simulink model "ex3_sim2m"  (R2022b)
settings: Solver=ode45  StartTime=0.0  StopTime=5  MaxStep=0.0001  RelTol=1e-3
undefined symbols (not defined in the file): d0, denD, DiscIntNeverNeededParam, mot, numD, pid, r, rad2pulse, Ts, umax
settings Model: Creator=loren  LastModifiedBy=loren
settings DataIOCC: ReturnWorkspaceOutputs=off

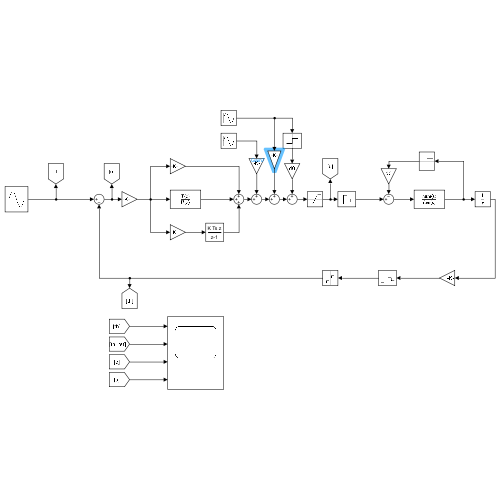
[thumbnail: Simulink's stored preview of the top-level diagram]
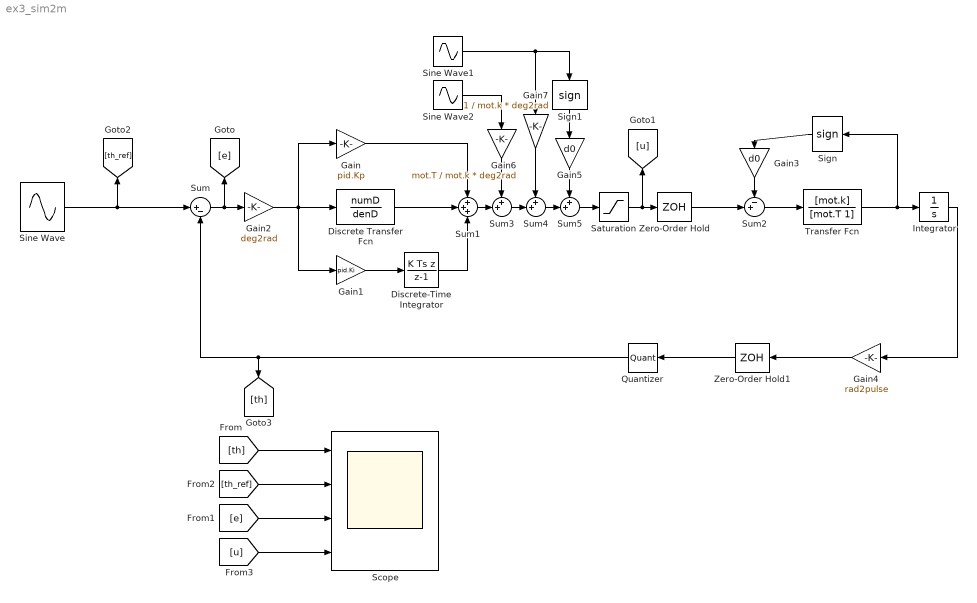
== system ex3_sim2m ==
  Discrete Transfer Fcn : DiscreteTransferFcn  Numerator=numD  Denominator=denD  SampleTime=Ts
  Discrete-Time Integrator : DiscreteIntegrator  IntegratorMethod=Integration: Backward Euler  SampleTime=Ts  ICPrevOutput=DiscIntNeverNeededParam  ICPrevScaledInput=DiscIntNeverNeededParam
  Gain : Gain  Gain=pid.Kp
  Gain1 : Gain  Gain=pid.Ki
  Gain2 : Gain  Gain=deg2rad
  Gain3 : Gain  Gain=d0
  Gain4 : Gain  Gain=rad2pulse
  Gain5 : Gain  Gain=d0
  Gain6 : Gain  Gain=mot.T / mot.k * deg2rad
  Gain7 : Gain  Gain=1 / mot.k * deg2rad
  Integrator : Integrator
  Quantizer : Quantizer  QuantizationInterval=pulse2deg
  Saturation : Saturate  UpperLimit=umax  LowerLimit=-umax
  Scope : Scope  NumInputPorts=4
  Sign : Signum  ZeroCross=off
  Sign1 : Signum  ZeroCross=off
  Sine Wave : Sin  Amplitude=r.A  Frequency=r.w  SampleTime=0
  Sine Wave1 : Sin  Amplitude=r.A * r.w  Frequency=r.w  Phase=pi / 2  SampleTime=0
  Sine Wave2 : Sin  Amplitude=-r.A * r.w^2  Frequency=r.w  SampleTime=0
  Sum : Sum  Inputs=|+-
  Sum1 : Sum  Inputs=+++
  Sum2 : Sum  Inputs=-+|
  Sum3 : Sum  Inputs=++|
  Sum4 : Sum  Inputs=++|
  Sum5 : Sum  Inputs=++|
  Transfer Fcn : TransferFcn  Numerator=[mot.k]  Denominator=[mot.T 1]
  Zero-Order Hold : ZeroOrderHold  SampleTime=Ts
  Zero-Order Hold1 : ZeroOrderHold  SampleTime=Ts
  wires:
  Gain1/1 -> Discrete-Time Integrator/1
  Sum/1 -> [e], Gain2/1
  Sine Wave/1 -> [th_ref], Sum/1
  Discrete Transfer Fcn/1 -> Sum1/2
  Discrete-Time Integrator/1 -> Sum1/3
  Gain/1 -> Sum1/1
  Saturation/1 -> Zero-Order Hold/1, [u]
  Transfer Fcn/1 -> Sign/1, Integrator/1
  Zero-Order Hold/1 -> Sum2/2
  Sum2/1 -> Transfer Fcn/1
  Zero-Order Hold1/1 -> Quantizer/1
  Quantizer/1 -> [th], Sum/2
  Gain2/1 -> Gain1/1, Gain/1, Discrete Transfer Fcn/1
  [th] -> Scope/1
  [th_ref] -> Scope/2
  [e] -> Scope/3
  [u] -> Scope/4
  Sign/1 -> Gain3/1
  Gain3/1 -> Sum2/1
  Integrator/1 -> Gain4/1
  Gain4/1 -> Zero-Order Hold1/1
  Sum3/1 -> Sum4/2
  Sum1/1 -> Sum3/2
  Sum4/1 -> Sum5/2
  Sum5/1 -> Saturation/1
  Sign1/1 -> Gain5/1
  Gain5/1 -> Sum5/1
  Gain6/1 -> Sum3/1
  Gain7/1 -> Sum4/1
  Sine Wave2/1 -> Gain6/1
  Sine Wave1/1 -> Gain7/1, Sign1/1
